simulink model "ngmresModel"  (R2020a)
settings: Solver=VariableStepAuto  StartTime=0.0  StopTime=10.0  RelTol=1e-3
values from neighbouring files (symbols this model uses):
  Ts = 1e-3    (= 0.001)    [runScript.m]
  u0 = u    [runScript.m]
  x0 = x    [runScript.m]
libraries: mympclib x1
settings Model: Creator=kohei  LastModifiedBy=kohei

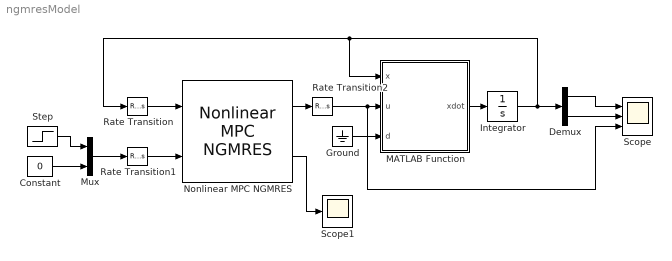
== system ngmresModel ==
  Constant : Constant  Value=0
  Demux : Demux  Outputs=2
  Ground : Ground
  Integrator : Integrator  InitialCondition=x0
  MATLAB Function : MATLAB Function  TreatAsAtomicUnit=on
  Mux : Mux  Inputs=2
  Nonlinear MPC NGMRES : mympclib/Nonlinear MPC NGMRES  params=params  nx=2  nmv=1  ns=1  nL=1  Ts=Ts  enableDist=off  nd=1  enableYseq=off  enableFnorm=on
      settings: SourceProductName=My MPC Library
  Rate Transition : RateTransition
  Rate Transition1 : RateTransition
  Rate Transition2 : RateTransition  InitialCondition=u0(1)
  Scope : Scope  NumInputPorts=3
  Scope1 : Scope
  Step : Step  After=2  SampleTime=0
  wires:
  Ground/1 -> MATLAB Function/3(d)
  MATLAB Function/1(xdot) -> Integrator/1
  Integrator/1 -> Demux/1, Rate Transition/1, MATLAB Function/1(x)
  Mux/1 -> Rate Transition1/1
  Constant/1 -> Mux/2
  Step/1 -> Mux/1
  Demux/1 -> Scope/1
  Demux/2 -> Scope/2
  Rate Transition/1 -> Nonlinear MPC NGMRES/1
  Rate Transition1/1 -> Nonlinear MPC NGMRES/2
  Rate Transition2/1 -> Scope/3, MATLAB Function/2(u)
  Nonlinear MPC NGMRES/2 -> Scope1/1
  Nonlinear MPC NGMRES/1 -> Rate Transition2/1

== matlab function ngmresModel/MATLAB Function ==
  data: x input; u input; xdot output; d input
function xdot = fcn(x,u,d)
xdot = statefcn(x,u,d);
end
